simulink model "RigidCompliance2015"  (R2015b)
settings: Solver=ode4  StartTime=0.0  StopTime=50  FixedStep=0.001  RelTol=1e-3
InitFcn:
  | %%%%%%%%%%%%%%%%%%%%%%%%%%% Robot's initial
  | %Initial position of robot
  | %q_0 = [-0.706;0.4326;0.9182;-1.696;-77.63;-1.726;0.2022];
  | %T_0 = [0.7508 -4063 0.5208 -0.4738;0.3266 -0.457 -0.8273 -8.688e-06;0.5741 0.7913 -0.2104 0.5303;0 0 0 1];
  | %For the case robot wants to make a circular behavior
  | q_0 = [0;0;0;-pi/2;0;0;0];
  | %T_0 = [0 0 -1 -0.39;0 1 0 0;1 0 0 0.71;0 0 0 1];
  | %Robot is in space
  | %q_0 = [-0.2434;0.3863;0.317;-1.6;-37.54;-1.032;0.06408];
  | 
  | 
  | %%%%%%%%%%%%%%%%%%%%%%%%%%% Impedance Controller
  | %Desired position of robot
  | T_des = [-0.3827 0 -0.9239 -0.5134;0 1 0 0;0.9239 0 -0.3827 0.5303;0 0 0 1];
  | %q_d = [0;pi/8;0;-pi/2;0;0;0]; starting point of the circle
  | 
  | %Proportional gains of compliance controller
  | K_x = [1500;1500;1500;200;200;200];
  | 
  | %Derivative gains of compliance controller
  | D_x =[500;150;500;100;100;100];
  | 
  | 
  | 
  | %%%%%%%%%%%%%%%%%%%%%%%%%%% Force Controller
  | %Desired force of EE
  | F_des = [1;zeros(5,1)];
  | 
  | %Proportional gains of force controller
  | K_f = [10;10;10;10;10;10];
  | 
  | %Derivative gains of force controller
  | D_f = [1;1;1;1;1;1];
  | 
  | %Integral gains of force cotroller
  | I_f = [40;40;40;40;40;40];
  | 
  | 
  | 
  | %%%%%%%%%%%%%%%%%%%%%%%%%%% Wall
  | %Parameters of wall plane: ax+by+cz
  | Pl_w = [1;0;0];
  | 
  | %Wall stiffness
  | K_w = [250;0;0];
  | % the stiffness is only in x direction of the wall, to make the circular behavior more realistic
  | 
  | %Wall first offset
  | d1 = -0.45;
  | 
  | %Wall second position
  | d2 = -10;
  | 
  | 
  | 
  | %%%%%%%%%%%%%%%%%%%%%%%%%%% Load
  | %Mass of the load
  | m_EE = 0;
  | 
  | %Position of the load
  | rCEE = zeros(3,1);
  | 
  | %T matrix for the load
  | TCP_T_EE = eye(4);
libraries: lwr_dynamics x5
settings Model: Creator=shahriari  LastModifiedBy=shahriari
settings DataIOCC: LimitDataPoints=off
settings DebuggingCC: AllowSymbolicDim=on
settings ModelReferenceCC: PropagateSignalLabelsOutOfModel=on
settings GRTTargetCC: GeneratePreprocessorConditionals=Disable all

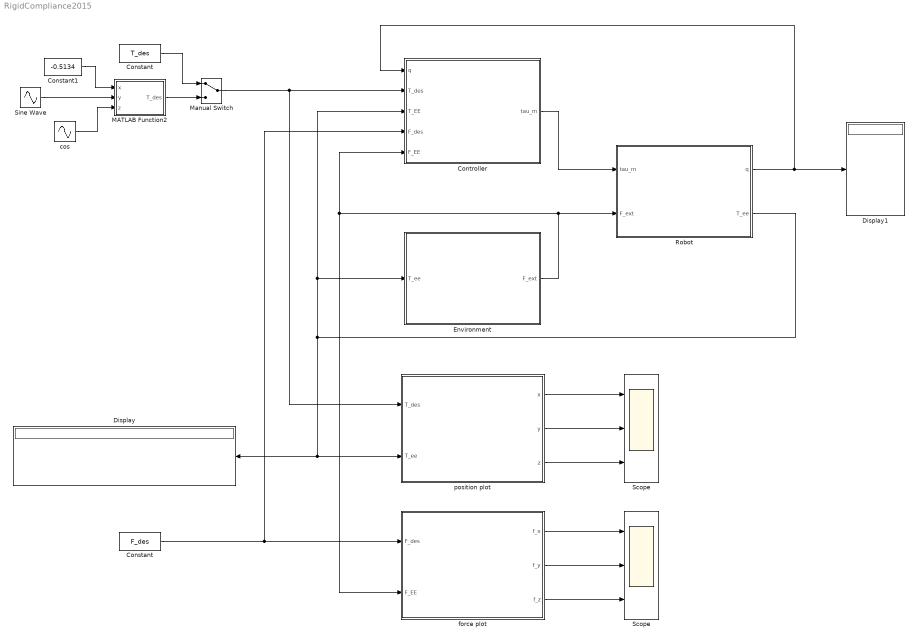
== system RigidCompliance2015 ==
  Constant : Constant  Value=T_des
  "Constant  " : Constant  Value=F_des
  Constant1 : Constant  Value=-0.5134
  Controller : Subsystem
  Display : Display
  Display1 : Display
  Environment : Subsystem
  MATLAB Function2 : MATLAB Function  TreatAsAtomicUnit=on
      settings: PermitHierarchicalResolution=ParametersOnly
  Manual Switch : ManualSwitch
  Robot : Subsystem
  Scope : Scope  NumInputPorts=3
  "Scope " : Scope  NumInputPorts=3
  Sine Wave : Sin  Amplitude=0.1492  Frequency=0.01  SampleTime=0
  cos : Sin  Amplitude=-0.1492  Bias=0.6795  Frequency=0.01  Phase=pi/2  SampleTime=0
  force plot : Subsystem
  position plot : Subsystem
  wires:
  Controller/1(tau_m) -> Robot/1(tau_m)
  Robot/2(T_ee) -> position plot/2(T_ee), Display/1, Environment/1(T_ee), Controller/3(T_EE)
  Environment/1(F_ext) -> force plot/2(F_EE), Controller/5(F_EE), Robot/2(F_ext)
  Robot/1(q) -> Controller/1(q), Display1/1
  Manual Switch/1 -> position plot/1(T_des), Controller/2(T_des)
  MATLAB Function2/1(T_des) -> Manual Switch/2
  Constant/1 -> Manual Switch/1
  Constant1/1 -> MATLAB Function2/1(x)
  Sine Wave/1 -> MATLAB Function2/2(y)
  cos/1 -> MATLAB Function2/3(z)
  "Constant  "/1 -> Controller/4(F_des), force plot/1(F_des)
  position plot/2(y) -> Scope/2
  position plot/3(z) -> Scope/3
  position plot/1(x) -> Scope/1
  force plot/2(f_y) -> "Scope "/2
  force plot/3(f_z) -> "Scope "/3
  force plot/1(f_x) -> "Scope "/1

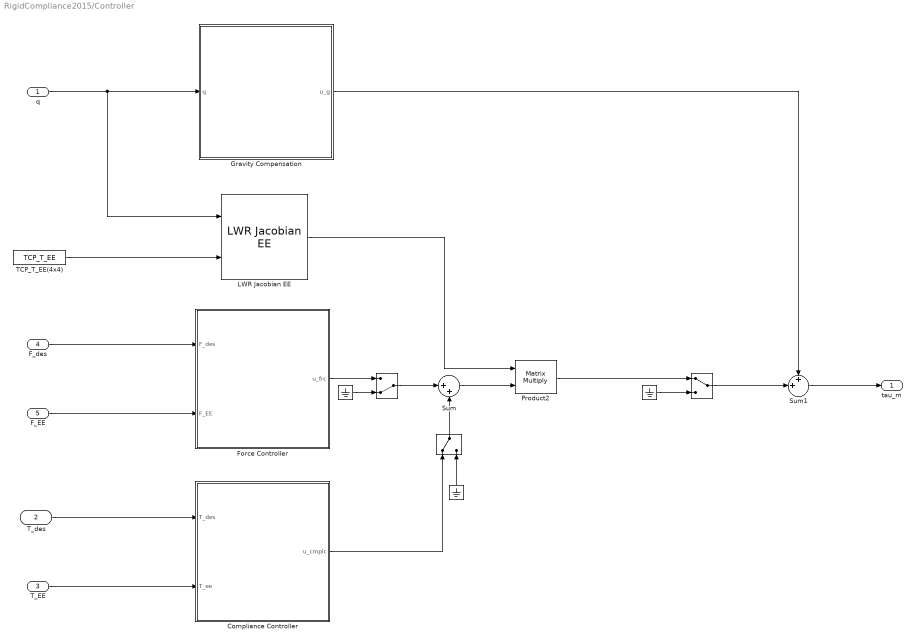
== system RigidCompliance2015/Controller ==
  q : Inport
  T_des : Inport  Port=2
  T_EE : Inport  Port=3
  F_des : Inport  Port=4
  F_EE : Inport  Port=5
  " " : Ground
  "  " : ManualSwitch
  "   " : ManualSwitch  CurrentSetting=0
  "    " : Ground
  "     " : Ground
  "      " : ManualSwitch
  Compliance Controller : Subsystem
  Force Controller : Subsystem
  Gravity Compensation : Subsystem
  LWR Jacobian EE : lwr_dynamics/Kinematics/LWR Jacobian EE
  Product2 : Product  Multiplication=Matrix(*)
  Sum : Sum  Inputs=|++
  Sum1 : Sum  Inputs=++|
  TCP_T_EE(4x4) : Constant  Value=TCP_T_EE
  tau_m : Outport
  wires:
  Sum1/1 -> tau_m/1
  T_EE/1 -> Compliance Controller/2(T_ee)
  T_des/1 -> Compliance Controller/1(T_des)
  Gravity Compensation/1(u_g) -> Sum1/1
  TCP_T_EE(4x4)/1 -> LWR Jacobian EE/2
  q/1 -> LWR Jacobian EE/1, Gravity Compensation/1(q)
  Sum/1 -> Product2/2
  LWR Jacobian EE/1 -> Product2/1
  F_des/1 -> Force Controller/1(F_des)
  F_EE/1 -> Force Controller/2(F_EE)
  "      "/1 -> Sum1/2
  "     "/1 -> "      "/2
  Force Controller/1(" u_frc") -> "   "/1
  "   "/1 -> Sum/1
  Compliance Controller/1(" u_cmplc") -> "  "/1
  "    "/1 -> "   "/2
  " "/1 -> "  "/2
  "  "/1 -> Sum/2
  Product2/1 -> "      "/1

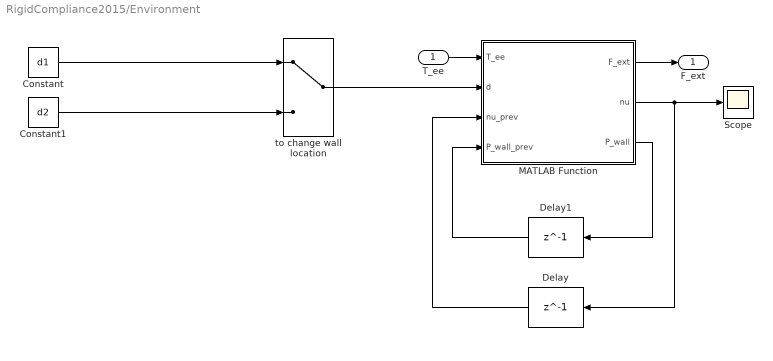
== system RigidCompliance2015/Environment ==
  T_ee : Inport
  Constant : Constant  Value=d1
  Constant1 : Constant  Value=d2
  Delay : Delay  DelayLength=1  InitialCondition=0  UseCircularBuffer=on
  Delay1 : Delay  DelayLength=1  InitialCondition=zeros(3,1)  UseCircularBuffer=on
  MATLAB Function : MATLAB Function  TreatAsAtomicUnit=on
      settings: PermitHierarchicalResolution=ParametersOnly
  Scope : Scope
  to change wall location : ManualSwitch
  F_ext : Outport
  wires:
  to change wall location/1 -> MATLAB Function/2(d)
  Constant/1 -> to change wall location/1
  Constant1/1 -> to change wall location/2
  MATLAB Function/1(F_ext) -> F_ext/1
  Delay/1 -> MATLAB Function/3(nu_prev)
  MATLAB Function/3(P_wall) -> Delay1/1
  Delay1/1 -> MATLAB Function/4(P_wall_prev)
  T_ee/1 -> MATLAB Function/1(T_ee)
  MATLAB Function/2(nu) -> Scope/1, Delay/1

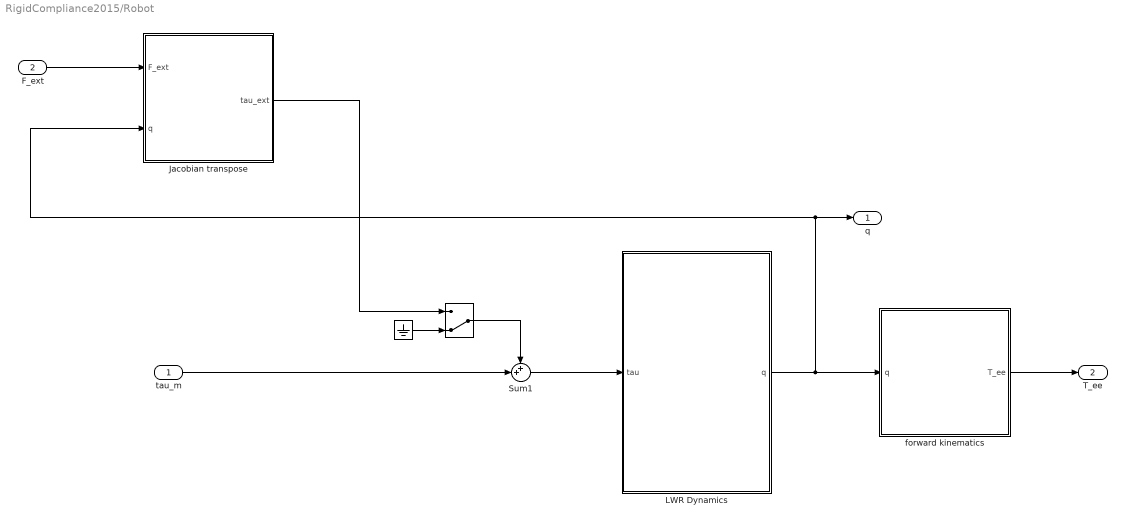
== system RigidCompliance2015/Robot ==
  tau_m : Inport
  F_ext : Inport  Port=2
  " " : ManualSwitch  CurrentSetting=0
  "  " : Ground
  Jacobian transpose : Subsystem
  LWR Dynamics : Subsystem
  Sum1 : Sum  Inputs=++|
  forward kinematics : Subsystem
  q : Outport
  T_ee : Outport  Port=2
  wires:
  Sum1/1 -> LWR Dynamics/1(tau)
  LWR Dynamics/1(q) -> Jacobian transpose/2(q), q/1, forward kinematics/1(q)
  forward kinematics/1("T_ee ") -> T_ee/1
  F_ext/1 -> Jacobian transpose/1(F_ext)
  Jacobian transpose/1(tau_ext) -> " "/1
  tau_m/1 -> Sum1/2
  "  "/1 -> " "/2
  " "/1 -> Sum1/1

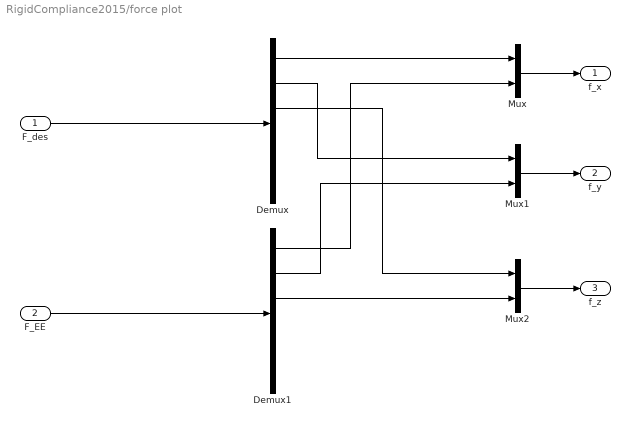
== system RigidCompliance2015/force plot ==
  F_des : Inport
  F_EE : Inport  Port=2
  Demux : Demux  Outputs=6
  Demux1 : Demux  Outputs=6
  Mux : Mux  Inputs=2
  Mux1 : Mux  Inputs=2
  Mux2 : Mux  Inputs=2
  f_x : Outport
  f_y : Outport  Port=2
  f_z : Outport  Port=3
  wires:
  F_des/1 -> Demux/1
  F_EE/1 -> Demux1/1
  Demux/1 -> Mux/1
  Demux1/1 -> Mux/2
  Mux2/1 -> f_z/1
  Mux1/1 -> f_y/1
  Mux/1 -> f_x/1
  Demux/2 -> Mux1/1
  Demux1/2 -> Mux1/2
  Demux/3 -> Mux2/1
  Demux1/3 -> Mux2/2

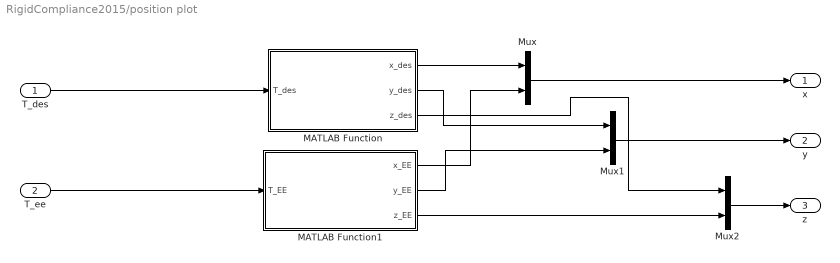
== system RigidCompliance2015/position plot ==
  T_des : Inport
  T_ee : Inport  Port=2
  MATLAB Function : MATLAB Function  TreatAsAtomicUnit=on
      settings: PermitHierarchicalResolution=ParametersOnly
  MATLAB Function1 : MATLAB Function  TreatAsAtomicUnit=on
      settings: PermitHierarchicalResolution=ParametersOnly
  Mux : Mux  Inputs=2
  Mux1 : Mux  Inputs=2
  Mux2 : Mux  Inputs=2
  x : Outport
  y : Outport  Port=2
  z : Outport  Port=3
  wires:
  T_des/1 -> MATLAB Function/1(T_des)
  T_ee/1 -> MATLAB Function1/1(T_EE)
  MATLAB Function/1(x_des) -> Mux/1
  MATLAB Function1/1(x_EE) -> Mux/2
  MATLAB Function/2(y_des) -> Mux1/1
  MATLAB Function1/2(y_EE) -> Mux1/2
  MATLAB Function/3(z_des) -> Mux2/1
  MATLAB Function1/3(z_EE) -> Mux2/2
  Mux2/1 -> z/1
  Mux1/1 -> y/1
  Mux/1 -> x/1

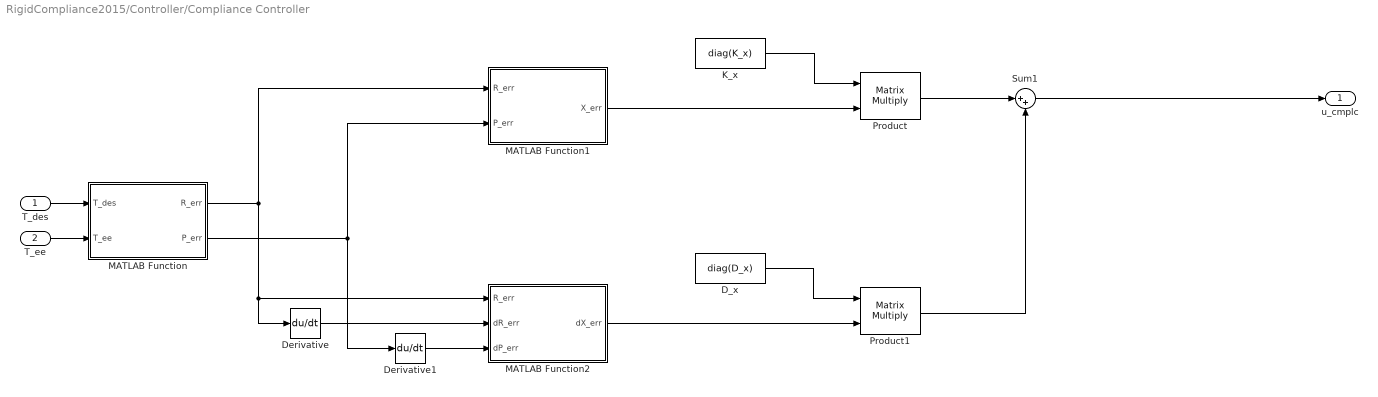
== system RigidCompliance2015/Controller/Compliance Controller ==
  T_des : Inport
  T_ee : Inport  Port=2
  D_x : Constant  Value=diag(D_x)
  Derivative : Derivative
  Derivative1 : Derivative
  K_x : Constant  Value=diag(K_x)
  MATLAB Function : MATLAB Function  TreatAsAtomicUnit=on
      settings: PermitHierarchicalResolution=ParametersOnly
  MATLAB Function1 : MATLAB Function  TreatAsAtomicUnit=on
      settings: PermitHierarchicalResolution=ParametersOnly
  MATLAB Function2 : MATLAB Function  TreatAsAtomicUnit=on
      settings: PermitHierarchicalResolution=ParametersOnly
  Product : Product  Multiplication=Matrix(*)
  Product1 : Product  Multiplication=Matrix(*)
  Sum1 : Sum  Inputs=|++
  " u_cmplc" : Outport
  wires:
  K_x/1 -> Product/1
  D_x/1 -> Product1/1
  Product/1 -> Sum1/1
  Product1/1 -> Sum1/2
  MATLAB Function1/1(X_err) -> Product/2
  T_des/1 -> MATLAB Function/1(T_des)
  T_ee/1 -> MATLAB Function/2(T_ee)
  MATLAB Function/1(R_err) -> MATLAB Function1/1(R_err), MATLAB Function2/1(R_err), Derivative/1
  MATLAB Function/2(P_err) -> MATLAB Function1/2(P_err), Derivative1/1
  Derivative/1 -> MATLAB Function2/2(dR_err)
  Derivative1/1 -> MATLAB Function2/3(dP_err)
  MATLAB Function2/1(dX_err) -> Product1/2
  Sum1/1 -> " u_cmplc"/1

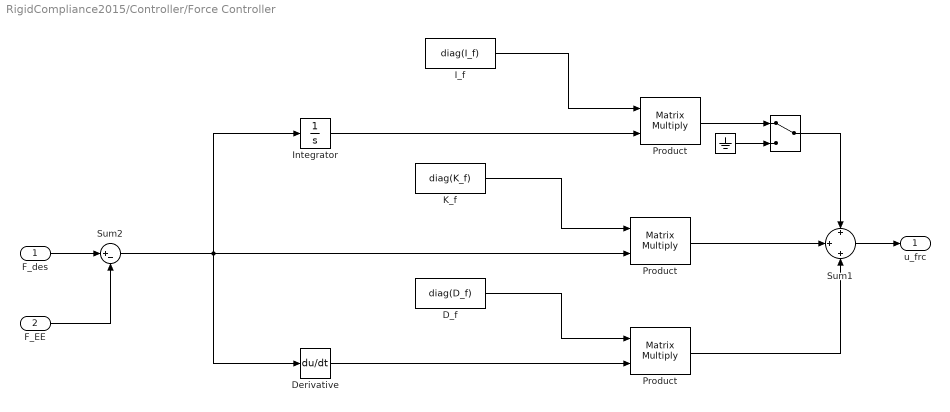
== system RigidCompliance2015/Controller/Force Controller ==
  F_des : Inport
  F_EE : Inport  Port=2
  "   " : ManualSwitch
  "    " : Ground
  D_f : Constant  Value=diag(D_f)
  Derivative : Derivative
  I_f : Constant  Value=diag(I_f)
  Integrator : Integrator
  K_f : Constant  Value=diag(K_f)
  Product : Product  Multiplication=Matrix(*)
  "Product " : Product  Multiplication=Matrix(*)
  "Product  " : Product  Multiplication=Matrix(*)
  Sum1 : Sum  Inputs=+|+|+
  Sum2 : Sum  Inputs=|+-
  " u_frc" : Outport
  wires:
  K_f/1 -> Product/1
  D_f/1 -> "Product  "/1
  F_des/1 -> Sum2/1
  F_EE/1 -> Sum2/2
  Derivative/1 -> "Product  "/2
  Sum1/1 -> " u_frc"/1
  "Product  "/1 -> Sum1/3
  Product/1 -> Sum1/2
  I_f/1 -> "Product "/1
  Sum2/1 -> Derivative/1, Product/2, Integrator/1
  Integrator/1 -> "Product "/2
  "Product "/1 -> "   "/1
  "   "/1 -> Sum1/1
  "    "/1 -> "   "/2

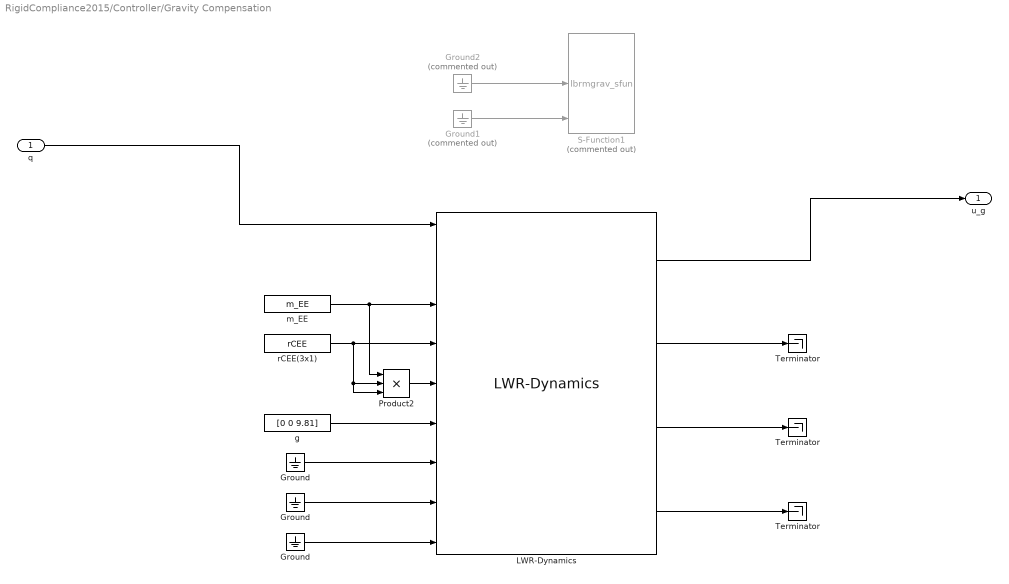
== system RigidCompliance2015/Controller/Gravity Compensation ==
  q : Inport
  Ground : Ground
  "Ground " : Ground
  "Ground  " : Ground
  Ground1 : Ground  Commented=on
  Ground2 : Ground  Commented=on
  LWR-Dynamics : lwr_dynamics/Dynamics/LWR-Dynamics
  Product2 : Product  Inputs=3  RndMeth=Zero
  S-Function1 : S-Function  Commented=on  FunctionName=lbrmgrav_sfun  SFunctionDeploymentMode=off  EnableBusSupport=off
  Terminator : Terminator
  "Terminator " : Terminator
  "Terminator  " : Terminator
  g : Constant  Value=[0 0 9.81]
  m_EE : Constant  Value=m_EE
  rCEE(3x1) : Constant  Value=rCEE
  u_g : Outport
  wires:
  Ground/1 -> LWR-Dynamics/7
  "Ground "/1 -> LWR-Dynamics/8
  "Ground  "/1 -> LWR-Dynamics/9
  g/1 -> LWR-Dynamics/6
  m_EE/1 -> LWR-Dynamics/3, Product2/1
  rCEE(3x1)/1 -> LWR-Dynamics/4, Product2/3, Product2/2
  Product2/1 -> LWR-Dynamics/5
  LWR-Dynamics/2 -> Terminator/1
  LWR-Dynamics/3 -> "Terminator "/1
  LWR-Dynamics/4 -> "Terminator  "/1
  Ground1/1 -> S-Function1/3
  Ground2/1 -> S-Function1/2
  q/1 -> LWR-Dynamics/1
  LWR-Dynamics/1 -> u_g/1

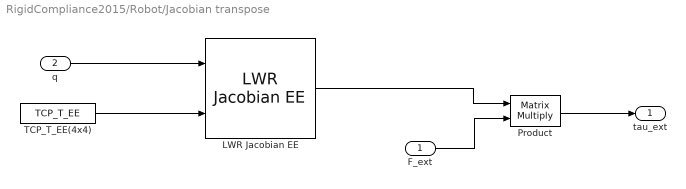
== system RigidCompliance2015/Robot/Jacobian transpose ==
  F_ext : Inport
  q : Inport  Port=2
  LWR Jacobian EE : lwr_dynamics/Kinematics/LWR Jacobian EE
  Product : Product  Multiplication=Matrix(*)
  TCP_T_EE(4x4) : Constant  Value=TCP_T_EE
  tau_ext : Outport
  wires:
  q/1 -> LWR Jacobian EE/1
  TCP_T_EE(4x4)/1 -> LWR Jacobian EE/2
  Product/1 -> tau_ext/1
  F_ext/1 -> Product/2
  LWR Jacobian EE/1 -> Product/1

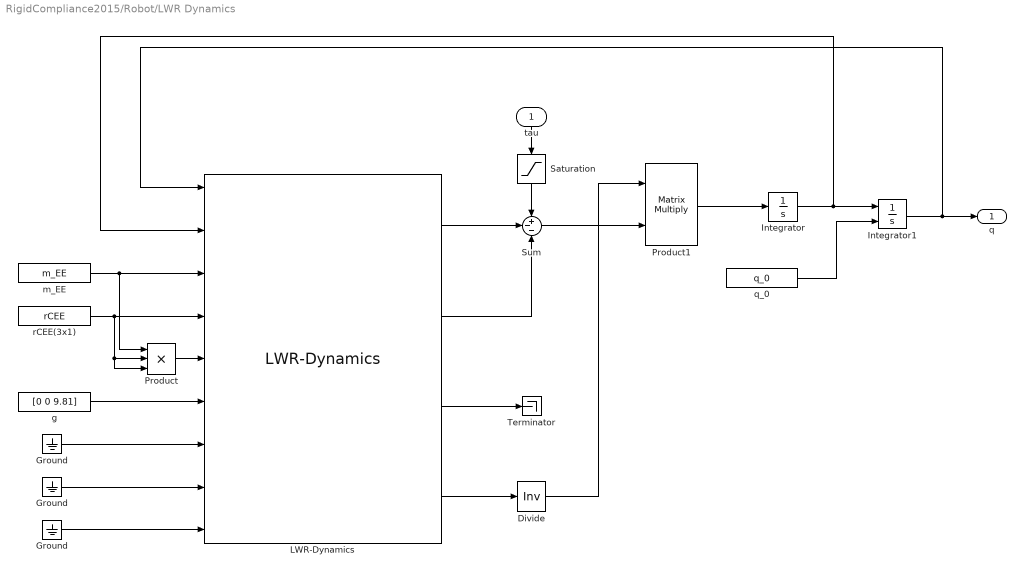
== system RigidCompliance2015/Robot/LWR Dynamics ==
  tau : Inport
  Divide : Product  Inputs=/  Multiplication=Matrix(*)
  Ground : Ground
  "Ground " : Ground
  "Ground  " : Ground
  Integrator : Integrator  InitialCondition=zeros(7,1)
  Integrator1 : Integrator  InitialConditionSource=external
  LWR-Dynamics : lwr_dynamics/Dynamics/LWR-Dynamics
  Product : Product  Inputs=3  RndMeth=Zero
  Product1 : Product  Multiplication=Matrix(*)  RndMeth=Zero
  Saturation : Saturate  UpperLimit=30  LowerLimit=-30
  Sum : Sum  Inputs=+--
  Terminator : Terminator
  g : Constant  Value=[0 0 9.81]
  m_EE : Constant  Value=m_EE
  q_0 : Constant  Value=q_0
  rCEE(3x1) : Constant  Value=rCEE
  q : Outport
  wires:
  Ground/1 -> LWR-Dynamics/7
  "Ground "/1 -> LWR-Dynamics/8
  "Ground  "/1 -> LWR-Dynamics/9
  g/1 -> LWR-Dynamics/6
  m_EE/1 -> LWR-Dynamics/3, Product/1
  rCEE(3x1)/1 -> LWR-Dynamics/4, Product/3, Product/2
  Product/1 -> LWR-Dynamics/5
  LWR-Dynamics/3 -> Terminator/1
  LWR-Dynamics/4 -> Divide/1
  LWR-Dynamics/1 -> Sum/2
  LWR-Dynamics/2 -> Sum/3
  tau/1 -> Saturation/1
  Product1/1 -> Integrator/1
  Integrator/1 -> LWR-Dynamics/2, Integrator1/1
  q_0/1 -> Integrator1/2
  Integrator1/1 -> LWR-Dynamics/1, q/1
  Sum/1 -> Product1/2
  Divide/1 -> Product1/1
  Saturation/1 -> Sum/1

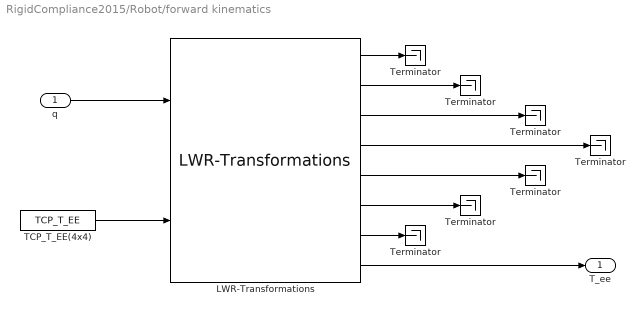
== system RigidCompliance2015/Robot/forward kinematics ==
  q : Inport
  LWR-Transformations : lwr_dynamics/Kinematics/LWR-Transformations
  TCP_T_EE(4x4) : Constant  Value=TCP_T_EE
  Terminator : Terminator
  "Terminator " : Terminator
  "Terminator  " : Terminator
  "Terminator   " : Terminator
  "Terminator    " : Terminator
  "Terminator     " : Terminator
  "Terminator      " : Terminator
  "T_ee " : Outport
  wires:
  TCP_T_EE(4x4)/1 -> LWR-Transformations/2
  q/1 -> LWR-Transformations/1
  LWR-Transformations/8 -> "T_ee "/1
  LWR-Transformations/1 -> Terminator/1
  LWR-Transformations/2 -> "Terminator "/1
  LWR-Transformations/3 -> "Terminator  "/1
  LWR-Transformations/4 -> "Terminator   "/1
  LWR-Transformations/5 -> "Terminator    "/1
  LWR-Transformations/6 -> "Terminator     "/1
  LWR-Transformations/7 -> "Terminator      "/1

== matlab function RigidCompliance2015/Environment/MATLAB Function ==
  data: T_ee input; F_ext output; d input; Pl_w parameter; K_w parameter; nu_prev input; nu output; P_wall_prev input; P_wall output
function [F_ext,nu,P_wall] = fcn(T_ee,d, Pl_w, K_w, nu_prev, P_wall_prev)
%#codegen

P_ee = T_ee(1:3,4);


if abs(Pl_w'*P_ee) < abs(d)
    nu = 0;
    P_wall = zeros(3,1);
    F_ext = zeros(6,1);
elseif nu_prev == 0
    nu = 1;
    P_wall = P_ee;
    F_ext = zeros(6,1);
else P_wall = P_wall_prev;
     F_ext = abs([diag(K_w)*(P_ee-P_wall);zeros(3,1)]);
     nu = 1;
end

== matlab function RigidCompliance2015/Controller/Compliance Controller/MATLAB Function ==
  data: T_des input; R_err output; T_ee input; P_err output
function [R_err, P_err] = fcn(T_des,T_ee)
%#codegen

R_err = T_ee(1:3,1:3)'*T_des(1:3,1:3);
P_err = T_des(1:3,4)-T_ee(1:3,4);

== matlab function RigidCompliance2015/Controller/Compliance Controller/MATLAB Function1 ==
  data: R_err input; X_err output; P_err input
function X_err  = fcn(R_err, P_err)
%#codegen

X_err = [P_err;zeros(3,1)];%rotm2eul(R_err)'];

== matlab function RigidCompliance2015/Controller/Compliance Controller/MATLAB Function2 ==
  data: R_err input; dX_err output; dR_err input; dP_err input
function dX_err  = fcn(R_err, dR_err, dP_err)
%#codegen

omega_str_err = dR_err*R_err';
dX_err = [dP_err;zeros(3,1)];%-omega_str_err(2,3);omega_str_err(1,3);-omega_str_err(1,2)];

== matlab function RigidCompliance2015/position plot/MATLAB Function ==
  data: x_des output; T_des input; y_des output; z_des output
function [x_des, y_des, z_des] = fcn(T_des)
%#codegen

x_des = T_des(1,4);
y_des = T_des(2,4);
z_des = T_des(3,4);

== matlab function RigidCompliance2015/position plot/MATLAB Function1 ==
  data: x_EE output; T_EE input; y_EE output; z_EE output
function [x_EE, y_EE, z_EE] = fcn(T_EE)
%#codegen

x_EE = T_EE(1,4);
y_EE = T_EE(2,4);
z_EE = T_EE(3,4);

== matlab function RigidCompliance2015/MATLAB Function2 ==
  data: x input; T_des output; y input; z input
function T_des = fcn(x,y,z)
%#codegen

T_des = [1 0 0 x;0 1 0 y;0 0 1 z;0 0 0 1];
